simulink model "NomotoModelTask12"  (R2015a)
settings: Solver=ode45  StartTime=0.0  StopTime=tstop  RelTol=1e-3
values from neighbouring files (symbols this model uses):
  amp = 0.3    [run_task_1_4.m]
  K = 0.8*(r(end)-r(1))/delta_step    [run_task_1_4.m]    (also in task_1_2.m = r_terminal/delta_c)
  omega_d = 0.008    [run_task_1_4.m]
  T = 59.13    [run_task_1_4.m]    (also in task_1_2.m = x(1))
  tsamp = 10    [run_task_1_4.m]
settings Model: Creator=ONL  LastModifiedBy=ONL

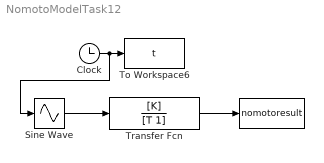
== system NomotoModelTask12 ==
  " " : ToWorkspace  VariableName=nomotoresult  SampleTime=-1
  Clock : Clock
  Sine Wave : Sin  TimeSource=Use external signal  Amplitude=-amp  Frequency=omega_d  SampleTime=0
  To Workspace6 : ToWorkspace  VariableName=t  SampleTime=tsamp
  Transfer Fcn : TransferFcn  Numerator=[K]  Denominator=[T 1]
  wires:
  Clock/1 -> Sine Wave/1, To Workspace6/1
  Sine Wave/1 -> Transfer Fcn/1
  Transfer Fcn/1 -> " "/1
